simulink model "ALL_JP360_DBW_V6_5_1103"  (R2022a)
settings: Solver=FixedStepAuto  StartTime=0.0  StopTime=inf  FixedStep=0.01  RelTol=1e-3  EnableMultiTasking=on
model workspace (MAT data in the model file):
  g = 9.8
undefined symbols (not defined in the file or in its folder): canChannel, delta_v_p, IPM_Line_C0, IPM_Line_C1, IPM_Line_C2, IPM_Line_C3, M, M_p, MRR_ObjDistX, MRR_ObjDistY, MRR_ObjFusionCamID, MRR_ObjFusionSig, MRR_ObjID, MRR_ObjRelVelX, MRR_ObjRelVelY, MRR_ObjType, MRR_ObjUpdFlg, none, obj_vaild, untracktime, V, videoinput
libraries: canfdmsglib x230, canfdlib x76, slpidlib x24, simulink x18, dspstat3 x14, ctrlSharedLib x1, simulink_extras x1, imaqlib x1, realtime_pacer_lib x1, dspvision x1, visionsinks x1
(part 11 of 55)

== system ALL_JP360_DBW_V6_5_1103/MsgFromCAN/CCAN_ADCU_MsgFromCAN/CCAN_ADCU_GW_EMS_Tq_0x101 ==
  CCAN_ADCU_GW_EMS_Tq_0x101FromInData : Inport  OutDataTypeStr=Bus:CAN_FD_MESSAGE_BUS
  Bus Creator : BusCreator  Inputs=7  OutDataTypeStr=Bus:CCAN_ADCU_GW_EMS_Tq_0x101  NonVirtualBus=on
  CAN FD Unpack : canfdmsglib/CAN FD Unpack  CANdbFile=HiFire_JPT360_CCAN_Matrix_CAN_V1.72_VP_ADCU.dbc  MsgList=(none)  MsgName=GW_EMS_Tq_0x101  ProtocolMode=CAN FD  MsgIDType=Standard (11-bit identifier)  MsgIdentifier=257  MsgLength=8  SignalInfo={'Checksum_0x101','56','8','BE','unsigned','Standard','0','1','0','0','255';'EMS_EngSpeed','33','15','BE','unsigned','Standard','0','0.5','0','0','16383';'EMS_EngSpeedError','32','1','BE','unsigned','Standard','0','1','0','0','1';'EMS_IndicatedRealEngTorq','16','12','BE','unsigned','Standard','0','0.5','-1000','-1000','1000';'EMS_RngModTorqCrSLeadMax','12','12','BE','unsigned','Standard','0','0.5','-1000','-1000','1000';'EMS_RngModTorqCrSLeadMin','52','12','BE','unsigned','Standard','0','0.5','-1000','-1000','1000';'RollingCounter_0x101','48','4','BE','unsigned','Standard','0','1','0','0','15'}  IDPort=off  TimestampPort=off  ErrorPort=off  RemotePort=off  LengthPort=off  StatusPort=off  BRSPort=off  ESIPort=off  DLCPort=off  ApplyMinMax=off
      settings: SourceProductBaseCode=XP,ME,VN  DataFormat=CANdb specified signals
  Data Type Conversion1 : DataTypeConversion  OutDataTypeStr=uint8  SaturateOnIntegerOverflow=off  RndMeth=Floor
  Data Type Conversion{2,4..6} (4 alike) : DataTypeConversion  OutDataTypeStr=single  SaturateOnIntegerOverflow=off  RndMeth=Floor
  Data Type Conversion3 : DataTypeConversion  OutDataTypeStr=boolean  SaturateOnIntegerOverflow=off  RndMeth=Floor
  Data Type Conversion7 : DataTypeConversion  OutDataTypeStr=int8  SaturateOnIntegerOverflow=off  RndMeth=Floor
  CCAN_ADCU_GW_EMS_Tq_0x101FromOutData : Outport  OutDataTypeStr=Bus:CCAN_ADCU_GW_EMS_Tq_0x101
  wires:
  CAN FD Unpack/1 -> Data Type Conversion1/1
  CAN FD Unpack/2 -> Data Type Conversion2/1
  CAN FD Unpack/3 -> Data Type Conversion3/1
  CAN FD Unpack/4 -> Data Type Conversion4/1
  CAN FD Unpack/5 -> Data Type Conversion5/1
  CAN FD Unpack/6 -> Data Type Conversion6/1
  CAN FD Unpack/7 -> Data Type Conversion7/1
  Data Type Conversion1/1 -> Bus Creator/1  "Checksum_0x101"
  Data Type Conversion2/1 -> Bus Creator/2  "EMS_EngSpeed"
  Data Type Conversion3/1 -> Bus Creator/3  "EMS_EngSpeedError"
  Data Type Conversion4/1 -> Bus Creator/4  "EMS_IndicatedRealEngTorq"
  Data Type Conversion5/1 -> Bus Creator/5  "EMS_RngModTorqCrSLeadMax"
  Data Type Conversion6/1 -> Bus Creator/6  "EMS_RngModTorqCrSLeadMin"
  Data Type Conversion7/1 -> Bus Creator/7  "RollingCounter_0x101"
  Bus Creator/1 -> CCAN_ADCU_GW_EMS_Tq_0x101FromOutData/1  "CCAN_ADCU_GW_EMS_Tq_0x101FromOutData"
  CCAN_ADCU_GW_EMS_Tq_0x101FromInData/1 -> CAN FD Unpack/1  "CCAN_ADCU_GW_EMS_Tq_0x101FromInData"

== system ALL_JP360_DBW_V6_5_1103/MsgFromCAN/CCAN_ADCU_MsgFromCAN/CCAN_ADCU_GW_EMS_WhlTq_0x107 ==
  CCAN_ADCU_GW_EMS_WhlTq_0x107FromInData : Inport  OutDataTypeStr=Bus:CAN_FD_MESSAGE_BUS
  Bus Creator : BusCreator  Inputs=9  OutDataTypeStr=Bus:CCAN_ADCU_GW_EMS_WhlTq_0x107  NonVirtualBus=on
  CAN FD Unpack : canfdmsglib/CAN FD Unpack  CANdbFile=HiFire_JPT360_CCAN_Matrix_CAN_V1.72_VP_ADCU.dbc  MsgList=(none)  MsgName=GW_EMS_WhlTq_0x107  ProtocolMode=CAN FD  MsgIDType=Standard (11-bit identifier)  MsgIdentifier=263  MsgLength=8  SignalInfo={'Checksum_0x107','56','8','BE','unsigned','Standard','0','1','0','0','255';'EMS_ACCPedalRatioError','53','1','BE','unsigned','Standard','0','1','0','0','1';'EMS_AccPedalRatio','40','8','BE','unsigned','Standard','0','0.3937','0','0','99.9998';'EMS_AccRAWPedalRatio','32','8','BE','unsigned','Standard','0','0.3937','0','0','99.9998';'EMS_BrkPedalStasus','54','2','BE','unsigned','Standard','0','1','0','0','3';'EMS_KickDown','52','1','BE','unsigned','Standard','0','1','0','0','1';'MaxIndicatedTorqWhl','8','16','BE','unsigned','Standard','0','1','-30000','-30000','30000';'MinIndicatedTorqWhl','24','16','BE','unsigned','Standard','0','1','-30000','-30000','30000';'RollingCounter_0x107','48','4','BE','unsigned','Standard','0','1','0','0','15'}  IDPort=off  TimestampPort=off  ErrorPort=off  RemotePort=off  LengthPort=off  StatusPort=off  BRSPort=off  ESIPort=off  DLCPort=off  ApplyMinMax=off
      settings: SourceProductBaseCode=XP,ME,VN  DataFormat=CANdb specified signals
  Data Type Conversion1 : DataTypeConversion  OutDataTypeStr=uint8  SaturateOnIntegerOverflow=off  RndMeth=Floor
  Data Type Conversion2 : DataTypeConversion  OutDataTypeStr=boolean  SaturateOnIntegerOverflow=off  RndMeth=Floor
  Data Type Conversion3 : DataTypeConversion  OutDataTypeStr=single  SaturateOnIntegerOverflow=off  RndMeth=Floor
  Data Type Conversion4 : DataTypeConversion  OutDataTypeStr=single  SaturateOnIntegerOverflow=off  RndMeth=Floor
  Data Type Conversion5 : DataTypeConversion  OutDataTypeStr=int8  SaturateOnIntegerOverflow=off  RndMeth=Floor
  Data Type Conversion6 : DataTypeConversion  OutDataTypeStr=boolean  SaturateOnIntegerOverflow=off  RndMeth=Floor
  Data Type Conversion7 : DataTypeConversion  OutDataTypeStr=int16  SaturateOnIntegerOverflow=off  RndMeth=Floor
  Data Type Conversion8 : DataTypeConversion  OutDataTypeStr=int16  SaturateOnIntegerOverflow=off  RndMeth=Floor
  Data Type Conversion9 : DataTypeConversion  OutDataTypeStr=int8  SaturateOnIntegerOverflow=off  RndMeth=Floor
  CCAN_ADCU_GW_EMS_WhlTq_0x107FromOutData : Outport  OutDataTypeStr=Bus:CCAN_ADCU_GW_EMS_WhlTq_0x107
  wires:
  CAN FD Unpack/1 -> Data Type Conversion1/1
  CAN FD Unpack/2 -> Data Type Conversion2/1
  CAN FD Unpack/3 -> Data Type Conversion3/1
  CAN FD Unpack/4 -> Data Type Conversion4/1
  CAN FD Unpack/5 -> Data Type Conversion5/1
  CAN FD Unpack/6 -> Data Type Conversion6/1
  CAN FD Unpack/7 -> Data Type Conversion7/1
  CAN FD Unpack/8 -> Data Type Conversion8/1
  CAN FD Unpack/9 -> Data Type Conversion9/1
  Data Type Conversion1/1 -> Bus Creator/1  "Checksum_0x107"
  Data Type Conversion2/1 -> Bus Creator/2  "EMS_ACCPedalRatioError"
  Data Type Conversion3/1 -> Bus Creator/3  "EMS_AccPedalRatio"
  Data Type Conversion4/1 -> Bus Creator/4  "EMS_AccRAWPedalRatio"
  Data Type Conversion5/1 -> Bus Creator/5  "EMS_BrkPedalStasus"
  Data Type Conversion6/1 -> Bus Creator/6  "EMS_KickDown"
  Data Type Conversion7/1 -> Bus Creator/7  "MaxIndicatedTorqWhl"
  Data Type Conversion8/1 -> Bus Creator/8  "MinIndicatedTorqWhl"
  Data Type Conversion9/1 -> Bus Creator/9  "RollingCounter_0x107"
  Bus Creator/1 -> CCAN_ADCU_GW_EMS_WhlTq_0x107FromOutData/1  "CCAN_ADCU_GW_EMS_WhlTq_0x107FromOutData"
  CCAN_ADCU_GW_EMS_WhlTq_0x107FromInData/1 -> CAN FD Unpack/1  "CCAN_ADCU_GW_EMS_WhlTq_0x107FromInData"

== system ALL_JP360_DBW_V6_5_1103/MsgFromCAN/CCAN_ADCU_MsgFromCAN/CCAN_ADCU_GW_IC_0x510 ==
  CCAN_ADCU_GW_IC_0x510FromInData : Inport  OutDataTypeStr=Bus:CAN_FD_MESSAGE_BUS
  Bus Creator : BusCreator  Inputs=11  OutDataTypeStr=Bus:CCAN_ADCU_GW_IC_0x510  NonVirtualBus=on
  CAN FD Unpack : canfdmsglib/CAN FD Unpack  CANdbFile=HiFire_JPT360_CCAN_Matrix_CAN_V1.72_VP_ADCU.dbc  MsgList=(none)  MsgName=GW_IC_0x510  ProtocolMode=CAN FD  MsgIDType=Standard (11-bit identifier)  MsgIdentifier=1296  MsgLength=8  SignalInfo={'Checksum_0x510','56','8','BE','unsigned','Standard','0','1','0','0','255';'IC_AirbagTelltaleBehavior','38','3','BE','unsigned','Standard','0','1','0','0','7';'IC_BrakeAirPressure','53','8','BE','unsigned','Standard','0','30','0','0','1200';'IC_CabLockSts','52','1','BE','unsigned','Standard','0','1','0','0','1';'IC_DISFail','29','1','BE','unsigned','Standard','0','1','0','0','1';'IC_OdometerMasterValue','16','24','BE','unsigned','Standard','0','0.1','0','0','999999';'IC_QDashACCFail','30','2','BE','unsigned','Standard','0','1','0','0','3';'IC_VehBrkPump_ERR_IC','28','1','BE','unsigned','Standard','0','1','0','0','1';'IC_VehSpd_HMI','45','9','BE','unsigned','Standard','0','1','0','0','500';'IC_tirelearning','25','3','BE','unsigned','Standard','0','1','0','0','8';'RollingCounter_0x510','48','4','BE','unsigned','Standard','0','1','0','0','15'}  IDPort=off  TimestampPort=off  ErrorPort=off  RemotePort=off  LengthPort=off  StatusPort=off  BRSPort=off  ESIPort=off  DLCPort=off  ApplyMinMax=off
      settings: SourceProductBaseCode=XP,ME,VN  DataFormat=CANdb specified signals
  Data Type Conversion1 : DataTypeConversion  OutDataTypeStr=uint8  SaturateOnIntegerOverflow=off  RndMeth=Floor
  Data Type Conversion{2,7,10..11} (4 alike) : DataTypeConversion  OutDataTypeStr=int8  SaturateOnIntegerOverflow=off  RndMeth=Floor
  Data Type Conversion3 : DataTypeConversion  OutDataTypeStr=int16  SaturateOnIntegerOverflow=off  RndMeth=Floor
  Data Type Conversion4 : DataTypeConversion  OutDataTypeStr=boolean  SaturateOnIntegerOverflow=off  RndMeth=Floor
  Data Type Conversion5 : DataTypeConversion  OutDataTypeStr=boolean  SaturateOnIntegerOverflow=off  RndMeth=Floor
  Data Type Conversion6 : DataTypeConversion  OutDataTypeStr=single  SaturateOnIntegerOverflow=off  RndMeth=Floor
  Data Type Conversion8 : DataTypeConversion  OutDataTypeStr=boolean  SaturateOnIntegerOverflow=off  RndMeth=Floor
  Data Type Conversion9 : DataTypeConversion  OutDataTypeStr=int16  SaturateOnIntegerOverflow=off  RndMeth=Floor
  CCAN_ADCU_GW_IC_0x510FromOutData : Outport  OutDataTypeStr=Bus:CCAN_ADCU_GW_IC_0x510
  wires:
  CAN FD Unpack/1 -> Data Type Conversion1/1
  CAN FD Unpack/2 -> Data Type Conversion2/1
  CAN FD Unpack/3 -> Data Type Conversion3/1
  CAN FD Unpack/4 -> Data Type Conversion4/1
  CAN FD Unpack/5 -> Data Type Conversion5/1
  CAN FD Unpack/6 -> Data Type Conversion6/1
  CAN FD Unpack/7 -> Data Type Conversion7/1
  CAN FD Unpack/8 -> Data Type Conversion8/1
  CAN FD Unpack/9 -> Data Type Conversion9/1
  CAN FD Unpack/10 -> Data Type Conversion10/1
  CAN FD Unpack/11 -> Data Type Conversion11/1
  Data Type Conversion1/1 -> Bus Creator/1  "Checksum_0x510"
  Data Type Conversion2/1 -> Bus Creator/2  "IC_AirbagTelltaleBehavior"
  Data Type Conversion3/1 -> Bus Creator/3  "IC_BrakeAirPressure"
  Data Type Conversion4/1 -> Bus Creator/4  "IC_CabLockSts"
  Data Type Conversion5/1 -> Bus Creator/5  "IC_DISFail"
  Data Type Conversion6/1 -> Bus Creator/6  "IC_OdometerMasterValue"
  Data Type Conversion7/1 -> Bus Creator/7  "IC_QDashACCFail"
  Data Type Conversion8/1 -> Bus Creator/8  "IC_VehBrkPump_ERR_IC"
  Data Type Conversion9/1 -> Bus Creator/9  "IC_VehSpd_HMI"
  Data Type Conversion10/1 -> Bus Creator/10  "IC_tirelearning"
  Data Type Conversion11/1 -> Bus Creator/11  "RollingCounter_0x510"
  Bus Creator/1 -> CCAN_ADCU_GW_IC_0x510FromOutData/1  "CCAN_ADCU_GW_IC_0x510FromOutData"
  CCAN_ADCU_GW_IC_0x510FromInData/1 -> CAN FD Unpack/1  "CCAN_ADCU_GW_IC_0x510FromInData"

== system ALL_JP360_DBW_V6_5_1103/MsgFromCAN/CCAN_ADCU_MsgFromCAN/CCAN_ADCU_GW_IC_Time_0x581 ==
  CCAN_ADCU_GW_IC_Time_0x581FromInData : Inport  OutDataTypeStr=Bus:CAN_FD_MESSAGE_BUS
  Bus Creator : BusCreator  Inputs=6  OutDataTypeStr=Bus:CCAN_ADCU_GW_IC_Time_0x581  NonVirtualBus=on
  CAN FD Unpack : canfdmsglib/CAN FD Unpack  CANdbFile=HiFire_JPT360_CCAN_Matrix_CAN_V1.72_VP_ADCU.dbc  MsgList=(none)  MsgName=GW_IC_Time_0x581  ProtocolMode=CAN FD  MsgIDType=Standard (11-bit identifier)  MsgIdentifier=1409  MsgLength=8  SignalInfo={'IC_Date','16','8','BE','unsigned','Standard','0','1','1','1','31';'IC_Hour','24','8','BE','unsigned','Standard','0','1','0','0','23';'IC_Minute','32','8','BE','unsigned','Standard','0','1','0','0','59';'IC_Month','8','8','BE','unsigned','Standard','0','1','1','1','12';'IC_Second','40','8','BE','unsigned','Standard','0','1','0','0','59';'IC_Year','0','8','BE','unsigned','Standard','0','1','2017','2017','2272'}  IDPort=off  TimestampPort=off  ErrorPort=off  RemotePort=off  LengthPort=off  StatusPort=off  BRSPort=off  ESIPort=off  DLCPort=off  ApplyMinMax=off
      settings: SourceProductBaseCode=XP,ME,VN  DataFormat=CANdb specified signals
  Data Type Conversion{1..5} (5 alike) : DataTypeConversion  OutDataTypeStr=int8  SaturateOnIntegerOverflow=off  RndMeth=Floor
  Data Type Conversion6 : DataTypeConversion  OutDataTypeStr=int16  SaturateOnIntegerOverflow=off  RndMeth=Floor
  CCAN_ADCU_GW_IC_Time_0x581FromOutData : Outport  OutDataTypeStr=Bus:CCAN_ADCU_GW_IC_Time_0x581
  wires:
  CAN FD Unpack/1 -> Data Type Conversion1/1
  CAN FD Unpack/2 -> Data Type Conversion2/1
  CAN FD Unpack/3 -> Data Type Conversion3/1
  CAN FD Unpack/4 -> Data Type Conversion4/1
  CAN FD Unpack/5 -> Data Type Conversion5/1
  CAN FD Unpack/6 -> Data Type Conversion6/1
  Data Type Conversion1/1 -> Bus Creator/1  "IC_Date"
  Data Type Conversion2/1 -> Bus Creator/2  "IC_Hour"
  Data Type Conversion3/1 -> Bus Creator/3  "IC_Minute"
  Data Type Conversion4/1 -> Bus Creator/4  "IC_Month"
  Data Type Conversion5/1 -> Bus Creator/5  "IC_Second"
  Data Type Conversion6/1 -> Bus Creator/6  "IC_Year"
  Bus Creator/1 -> CCAN_ADCU_GW_IC_Time_0x581FromOutData/1  "CCAN_ADCU_GW_IC_Time_0x581FromOutData"
  CCAN_ADCU_GW_IC_Time_0x581FromInData/1 -> CAN FD Unpack/1  "CCAN_ADCU_GW_IC_Time_0x581FromInData"

== system ALL_JP360_DBW_V6_5_1103/MsgFromCAN/CCAN_ADCU_MsgFromCAN/CCAN_ADCU_GW_MP5_0x530 ==
  CCAN_ADCU_GW_MP5_0x530FromInData : Inport  OutDataTypeStr=Bus:CAN_FD_MESSAGE_BUS
  Bus Creator : BusCreator  Inputs=42  OutDataTypeStr=Bus:CCAN_ADCU_GW_MP5_0x530  NonVirtualBus=on
  CAN FD Unpack : canfdmsglib/CAN FD Unpack  CANdbFile=HiFire_JPT360_CCAN_Matrix_CAN_V1.72_VP_ADCU.dbc  MsgList=(none)  MsgName=GW_MP5_0x530  ProtocolMode=CAN FD  MsgIDType=Standard (11-bit identifier)  MsgIdentifier=1328  MsgLength=8  SignalInfo={'IVI_Driving_mode_req','36','4','BE','unsigned','Standard','0','1','0','0','15';'IVI_EcallRq','27','1','BE','unsigned','Standard','0','1','0','0','1';'IVI_FlashFlag','35','1','BE','unsigned','Standard','0','1','0','0','1';'IVI_HDCSwitchSetting','24','1','BE','unsigned','Standard','0','1','0','0','1';'MP5_AEB_ON_OFF','12','1','BE','unsigned','Standard','0','1','0','0','1';'MP5_AFS_SwtichSts','16','1','BE','unsigned','Standard','0','1','0','0','1';'MP5_APA_Available_Sts','56','2','BE','unsigned','Standard','0','1','0','0','1';'MP5_AVM_Angle','2','4','BE','unsigned','Standard','0','1','0','0','15';'MP5_AVM_Button','6','2','BE','unsigned','Standard','0','1','0','0','3';'MP5_AVM_RotationChange','63','6','BE','unsigned','Standard','0','1','0','0','63';'MP5_AVM_RotationDirection','61','2','BE','unsigned','Standard','0','1','0','0','3';'MP5_AlarmOrNot','23','1','BE','unsigned','Standard','0','1','0','0','1';'MP5_AlarmStatus','21','2','BE','unsigned','Standard','0','1','0','0','3';'MP5_BSDLCA_Active','41','1','BE','unsigned','Standard','0','1','0','0','1';'MP5_BSDSoundSwitchSts','32','1','BE','unsigned','Standard','0','1','0','0','1';'MP5_BSDSwitchSts','15','1','BE','unsigned','Standard','0','1','0','0','1';'MP5_CST_ON_OFF','33','1','BE','unsigned','Standard','0','1','0','0','1';'MP5_ConnectivityReset','34','1','BE','unsigned','Standard','0','1','0','0','1';'MP5_DCLC_switchSts','30','1','BE','unsigned','Standard','0','1','0','0','1';'MP5_DDDMenuReq','42','1','BE','unsigned','Standard','0','1','0','0','1';'MP5_DOA_Active','55','1','BE','unsigned','Standard','0','1','0','0','1';'MP5_ELK_switchSts','29','1','BE','unsigned','Standard','0','1','0','0','1';'MP5_ESP_ON_OFF','8','1','BE','unsigned','Standard','0','1','0','0','1';'MP5_EmergencyTowingSetting','25','1','BE','unsigned','Standard','0','1','0','0','1';'MP5_FCW_ON_OFF','13','1','BE','unsigned','Standard','0','1','0','0','1';'MP5_FCW_Sensitive','0','2','BE','unsigned','Standard','0','1','0','0','3';'MP5_ICMenuActive_Button','19','2','BE','unsigned','Standard','0','1','0','0','3';'MP5_ICMenuShift_Button','10','2','BE','unsigned','Standard','0','1','0','0','3';'MP5_IHCMenuReq','53','1','BE','unsigned','Standard','0','1','0','0','1';'MP5_LAEB_switchSts','28','1','BE','unsigned','Standard','0','1','0','0','1';'MP5_LDWSensitvity','46','2','BE','unsigned','Standard','0','1','0','0','3';'MP5_LDWWarning','44','2','BE','unsigned','Standard','0','1','0','0','3';'MP5_LaneAssitTypeReq','17','2','BE','unsigned','Standard','0','1','0','0','3';'MP5_PaakReset_Req','31','1','BE','unsigned','Standard','0','1','0','0','1';'MP5_PrdeProt_ON_OFF','54','1','BE','unsigned','Standard','0','1','0','0','1';'MP5_RCTA_Active','40','1','BE','unsigned','Standard','0','1','0','0','1';'MP5_RCW_Active','26','1','BE','unsigned','Standard','0','1','0','0','1';'MP5_SDGSwitchSts','14','1','BE','unsigned','Standard','0','1','0','0','1';'MP5_TPMSAutoLocationSetting','58','1','BE','unsigned','Standard','0','1','0','0','1';'MP5_TSRMenuReq','43','1','BE','unsigned','Standard','0','1','0','0','1';'MP5_View_Choice','9','1','BE','unsigned','Standard','0','1','0','0','1';'MP5_VspVoiceTypeSetting','59','2','BE','unsigned','Standard','0','1','0','0','3'}  IDPort=off  TimestampPort=off  ErrorPort=off  RemotePort=off  LengthPort=off  StatusPort=off  BRSPort=off  ESIPort=off  DLCPort=off  ApplyMinMax=off
      settings: SourceProductBaseCode=XP,ME,VN  DataFormat=CANdb specified signals
  Data Type Conversion{1,7..11,13,26..28,31..33,42} (14 alike) : DataTypeConversion  OutDataTypeStr=int8  SaturateOnIntegerOverflow=off  RndMeth=Floor
  Data Type Conversion{2..6,12,14..25,29..30,34..41} (28 alike) : DataTypeConversion  OutDataTypeStr=boolean  SaturateOnIntegerOverflow=off  RndMeth=Floor
  CCAN_ADCU_GW_MP5_0x530FromOutData : Outport  OutDataTypeStr=Bus:CCAN_ADCU_GW_MP5_0x530
  wires:
  CAN FD Unpack/1 -> Data Type Conversion1/1
  CAN FD Unpack/2 -> Data Type Conversion2/1
  CAN FD Unpack/3 -> Data Type Conversion3/1
  CAN FD Unpack/4 -> Data Type Conversion4/1
  CAN FD Unpack/5 -> Data Type Conversion5/1
  CAN FD Unpack/6 -> Data Type Conversion6/1
  CAN FD Unpack/7 -> Data Type Conversion7/1
  CAN FD Unpack/8 -> Data Type Conversion8/1
  CAN FD Unpack/9 -> Data Type Conversion9/1
  CAN FD Unpack/10 -> Data Type Conversion10/1
  CAN FD Unpack/11 -> Data Type Conversion11/1
  CAN FD Unpack/12 -> Data Type Conversion12/1
  CAN FD Unpack/13 -> Data Type Conversion13/1
  CAN FD Unpack/14 -> Data Type Conversion14/1
  CAN FD Unpack/15 -> Data Type Conversion15/1
  CAN FD Unpack/16 -> Data Type Conversion16/1
  CAN FD Unpack/17 -> Data Type Conversion17/1
  CAN FD Unpack/18 -> Data Type Conversion18/1
  CAN FD Unpack/19 -> Data Type Conversion19/1
  CAN FD Unpack/20 -> Data Type Conversion20/1
  CAN FD Unpack/21 -> Data Type Conversion21/1
  CAN FD Unpack/22 -> Data Type Conversion22/1
  CAN FD Unpack/23 -> Data Type Conversion23/1
  CAN FD Unpack/24 -> Data Type Conversion24/1
  CAN FD Unpack/25 -> Data Type Conversion25/1
  CAN FD Unpack/26 -> Data Type Conversion26/1
  CAN FD Unpack/27 -> Data Type Conversion27/1
  CAN FD Unpack/28 -> Data Type Conversion28/1
  CAN FD Unpack/29 -> Data Type Conversion29/1
  CAN FD Unpack/30 -> Data Type Conversion30/1
  CAN FD Unpack/31 -> Data Type Conversion31/1
  CAN FD Unpack/32 -> Data Type Conversion32/1
  CAN FD Unpack/33 -> Data Type Conversion33/1
  CAN FD Unpack/34 -> Data Type Conversion34/1
  CAN FD Unpack/35 -> Data Type Conversion35/1
  CAN FD Unpack/36 -> Data Type Conversion36/1
  CAN FD Unpack/37 -> Data Type Conversion37/1
  CAN FD Unpack/38 -> Data Type Conversion38/1
  CAN FD Unpack/39 -> Data Type Conversion39/1
  CAN FD Unpack/40 -> Data Type Conversion40/1
  CAN FD Unpack/41 -> Data Type Conversion41/1
  CAN FD Unpack/42 -> Data Type Conversion42/1
  Data Type Conversion1/1 -> Bus Creator/1  "IVI_Driving_mode_req"
  Data Type Conversion2/1 -> Bus Creator/2  "IVI_EcallRq"
  Data Type Conversion3/1 -> Bus Creator/3  "IVI_FlashFlag"
  Data Type Conversion4/1 -> Bus Creator/4  "IVI_HDCSwitchSetting"
  Data Type Conversion5/1 -> Bus Creator/5  "MP5_AEB_ON_OFF"
  Data Type Conversion6/1 -> Bus Creator/6  "MP5_AFS_SwtichSts"
  Data Type Conversion7/1 -> Bus Creator/7  "MP5_APA_Available_Sts"
  Data Type Conversion8/1 -> Bus Creator/8  "MP5_AVM_Angle"
  Data Type Conversion9/1 -> Bus Creator/9  "MP5_AVM_Button"
  Data Type Conversion10/1 -> Bus Creator/10  "MP5_AVM_RotationChange"
  Data Type Conversion11/1 -> Bus Creator/11  "MP5_AVM_RotationDirection"
  Data Type Conversion12/1 -> Bus Creator/12  "MP5_AlarmOrNot"
  Data Type Conversion13/1 -> Bus Creator/13  "MP5_AlarmStatus"
  Data Type Conversion14/1 -> Bus Creator/14  "MP5_BSDLCA_Active"
  Data Type Conversion15/1 -> Bus Creator/15  "MP5_BSDSoundSwitchSts"
  Data Type Conversion16/1 -> Bus Creator/16  "MP5_BSDSwitchSts"
  Data Type Conversion17/1 -> Bus Creator/17  "MP5_CST_ON_OFF"
  Data Type Conversion18/1 -> Bus Creator/18  "MP5_ConnectivityReset"
  Data Type Conversion19/1 -> Bus Creator/19  "MP5_DCLC_switchSts"
  Data Type Conversion20/1 -> Bus Creator/20  "MP5_DDDMenuReq"
  Data Type Conversion21/1 -> Bus Creator/21  "MP5_DOA_Active"
  Data Type Conversion22/1 -> Bus Creator/22  "MP5_ELK_switchSts"
  Data Type Conversion23/1 -> Bus Creator/23  "MP5_ESP_ON_OFF"
  Data Type Conversion24/1 -> Bus Creator/24  "MP5_EmergencyTowingSetting"
  Data Type Conversion25/1 -> Bus Creator/25  "MP5_FCW_ON_OFF"
  Data Type Conversion26/1 -> Bus Creator/26  "MP5_FCW_Sensitive"
  Data Type Conversion27/1 -> Bus Creator/27  "MP5_ICMenuActive_Button"
  Data Type Conversion28/1 -> Bus Creator/28  "MP5_ICMenuShift_Button"
  Data Type Conversion29/1 -> Bus Creator/29  "MP5_IHCMenuReq"
  Data Type Conversion30/1 -> Bus Creator/30  "MP5_LAEB_switchSts"
  Data Type Conversion31/1 -> Bus Creator/31  "MP5_LDWSensitvity"
  Data Type Conversion32/1 -> Bus Creator/32  "MP5_LDWWarning"
  Data Type Conversion33/1 -> Bus Creator/33  "MP5_LaneAssitTypeReq"
  Data Type Conversion34/1 -> Bus Creator/34  "MP5_PaakReset_Req"
  Data Type Conversion35/1 -> Bus Creator/35  "MP5_PrdeProt_ON_OFF"
  Data Type Conversion36/1 -> Bus Creator/36  "MP5_RCTA_Active"
  Data Type Conversion37/1 -> Bus Creator/37  "MP5_RCW_Active"
  Data Type Conversion38/1 -> Bus Creator/38  "MP5_SDGSwitchSts"
  Data Type Conversion39/1 -> Bus Creator/39  "MP5_TPMSAutoLocationSetting"
  Data Type Conversion40/1 -> Bus Creator/40  "MP5_TSRMenuReq"
  Data Type Conversion41/1 -> Bus Creator/41  "MP5_View_Choice"
  Data Type Conversion42/1 -> Bus Creator/42  "MP5_VspVoiceTypeSetting"
  Bus Creator/1 -> CCAN_ADCU_GW_MP5_0x530FromOutData/1  "CCAN_ADCU_GW_MP5_0x530FromOutData"
  CCAN_ADCU_GW_MP5_0x530FromInData/1 -> CAN FD Unpack/1  "CCAN_ADCU_GW_MP5_0x530FromInData"

== system ALL_JP360_DBW_V6_5_1103/MsgFromCAN/CCAN_ADCU_MsgFromCAN/CCAN_ADCU_GW_MP5_AVM_0x3A1 ==
  CCAN_ADCU_GW_MP5_AVM_0x3A1FromInData : Inport  OutDataTypeStr=Bus:CAN_FD_MESSAGE_BUS
  Bus Creator : BusCreator  Inputs=8  OutDataTypeStr=Bus:CCAN_ADCU_GW_MP5_AVM_0x3A1  NonVirtualBus=on
  CAN FD Unpack : canfdmsglib/CAN FD Unpack  CANdbFile=HiFire_JPT360_CCAN_Matrix_CAN_V1.72_VP_ADCU.dbc  MsgList=(none)  MsgName=GW_MP5_AVM_0x3A1  ProtocolMode=CAN FD  MsgIDType=Standard (11-bit identifier)  MsgIdentifier=929  MsgLength=8  SignalInfo={'MP5_AVMAuxLineCtrl','14','2','BE','unsigned','Standard','0','1','0','0','3';'MP5_AVMBodyColor','10','4','BE','unsigned','Standard','0','1','0','0','15';'MP5_AVMCarHyalineCtrl','0','8','BE','unsigned','Standard','0','1','0','0','100';'MP5_AVMRGearDlyDisplay','8','2','BE','unsigned','Standard','0','1','0','0','3';'MP5_InterfaceChangeSingnal','51','3','BE','unsigned','Standard','0','1','0','0','7';'MP5_TrnLfMode','54','2','BE','unsigned','Standard','0','1','0','0','3';'MP5_Xlevel','24','16','BE','unsigned','Standard','0','1','0','0','65534';'MP5_Ylevel','40','16','BE','unsigned','Standard','0','1','0','0','65534'}  IDPort=off  TimestampPort=off  ErrorPort=off  RemotePort=off  LengthPort=off  StatusPort=off  BRSPort=off  ESIPort=off  DLCPort=off  ApplyMinMax=off
      settings: SourceProductBaseCode=XP,ME,VN  DataFormat=CANdb specified signals
  Data Type Conversion{1..6} (6 alike) : DataTypeConversion  OutDataTypeStr=int8  SaturateOnIntegerOverflow=off  RndMeth=Floor
  Data Type Conversion7 : DataTypeConversion  OutDataTypeStr=uint16  SaturateOnIntegerOverflow=off  RndMeth=Floor
  Data Type Conversion8 : DataTypeConversion  OutDataTypeStr=uint16  SaturateOnIntegerOverflow=off  RndMeth=Floor
  CCAN_ADCU_GW_MP5_AVM_0x3A1FromOutData : Outport  OutDataTypeStr=Bus:CCAN_ADCU_GW_MP5_AVM_0x3A1
  wires:
  CAN FD Unpack/1 -> Data Type Conversion1/1
  CAN FD Unpack/2 -> Data Type Conversion2/1
  CAN FD Unpack/3 -> Data Type Conversion3/1
  CAN FD Unpack/4 -> Data Type Conversion4/1
  CAN FD Unpack/5 -> Data Type Conversion5/1
  CAN FD Unpack/6 -> Data Type Conversion6/1
  CAN FD Unpack/7 -> Data Type Conversion7/1
  CAN FD Unpack/8 -> Data Type Conversion8/1
  Data Type Conversion1/1 -> Bus Creator/1  "MP5_AVMAuxLineCtrl"
  Data Type Conversion2/1 -> Bus Creator/2  "MP5_AVMBodyColor"
  Data Type Conversion3/1 -> Bus Creator/3  "MP5_AVMCarHyalineCtrl"
  Data Type Conversion4/1 -> Bus Creator/4  "MP5_AVMRGearDlyDisplay"
  Data Type Conversion5/1 -> Bus Creator/5  "MP5_InterfaceChangeSingnal"
  Data Type Conversion6/1 -> Bus Creator/6  "MP5_TrnLfMode"
  Data Type Conversion7/1 -> Bus Creator/7  "MP5_Xlevel"
  Data Type Conversion8/1 -> Bus Creator/8  "MP5_Ylevel"
  Bus Creator/1 -> CCAN_ADCU_GW_MP5_AVM_0x3A1FromOutData/1  "CCAN_ADCU_GW_MP5_AVM_0x3A1FromOutData"
  CCAN_ADCU_GW_MP5_AVM_0x3A1FromInData/1 -> CAN FD Unpack/1  "CCAN_ADCU_GW_MP5_AVM_0x3A1FromInData"

== system ALL_JP360_DBW_V6_5_1103/MsgFromCAN/CCAN_ADCU_MsgFromCAN/CCAN_ADCU_GW_MP5_LicensePlateNum_0x375 ==
  CCAN_ADCU_GW_MP5_LicensePlateNum_0x375FromInData : Inport  OutDataTypeStr=Bus:CAN_FD_MESSAGE_BUS
  Bus Creator : BusCreator  Inputs=1  OutDataTypeStr=Bus:CCAN_ADCU_GW_MP5_LicensePlateNum_0x375  NonVirtualBus=on
  CAN FD Unpack : canfdmsglib/CAN FD Unpack  CANdbFile=HiFire_JPT360_CCAN_Matrix_CAN_V1.72_VP_ADCU.dbc  MsgList=(none)  MsgName=GW_MP5_LicensePlateNum_0x375  ProtocolMode=CAN FD  MsgIDType=Standard (11-bit identifier)  MsgIdentifier=885  MsgLength=8  SignalInfo={'MP5_LicenseInfo','56','64','BE','unsigned','Standard','0','1','0','0','1.84467440737095e+19'}  IDPort=off  TimestampPort=off  ErrorPort=off  RemotePort=off  LengthPort=off  StatusPort=off  BRSPort=off  ESIPort=off  DLCPort=off  ApplyMinMax=off
      settings: SourceProductBaseCode=XP,ME,VN  DataFormat=CANdb specified signals
  Data Type Conversion1 : DataTypeConversion  OutDataTypeStr=uint64  SaturateOnIntegerOverflow=off  RndMeth=Floor
  CCAN_ADCU_GW_MP5_LicensePlateNum_0x375FromOutData : Outport  OutDataTypeStr=Bus:CCAN_ADCU_GW_MP5_LicensePlateNum_0x375
  wires:
  Data Type Conversion1/1 -> Bus Creator/1  "MP5_LicenseInfo"
  Bus Creator/1 -> CCAN_ADCU_GW_MP5_LicensePlateNum_0x375FromOutData/1  "CCAN_ADCU_GW_MP5_LicensePlateNum_0x375FromOutData"
  CCAN_ADCU_GW_MP5_LicensePlateNum_0x375FromInData/1 -> CAN FD Unpack/1  "CCAN_ADCU_GW_MP5_LicensePlateNum_0x375FromInData"

== system ALL_JP360_DBW_V6_5_1103/MsgFromCAN/CCAN_ADCU_MsgFromCAN/CCAN_ADCU_GW_MP5_NAV_0x533 ==
  CCAN_ADCU_GW_MP5_NAV_0x533FromInData : Inport  OutDataTypeStr=Bus:CAN_FD_MESSAGE_BUS
  Bus Creator : BusCreator  Inputs=17  OutDataTypeStr=Bus:CCAN_ADCU_GW_MP5_NAV_0x533  NonVirtualBus=on
  CAN FD Unpack : canfdmsglib/CAN FD Unpack  CANdbFile=HiFire_JPT360_CCAN_Matrix_CAN_V1.72_VP_ADCU.dbc  MsgList=(none)  MsgName=GW_MP5_NAV_0x533  ProtocolMode=CAN FD  MsgIDType=Standard (11-bit identifier)  MsgIdentifier=1331  MsgLength=8  SignalInfo={'IVI_APA_SelPrkOutDirReq','34','3','BE','unsigned','Standard','0','1','0','0','7';'MP5_APAActive_Cmd','26','1','BE','unsigned','Standard','0','1','0','0','1';'MP5_APA_ConfirmButton','27','2','BE','unsigned','Standard','0','1','0','0','3';'MP5_APA_Function_Select','37','3','BE','unsigned','Standard','0','1','0','0','7';'MP5_ContnPrkgReq','24','2','BE','unsigned','Standard','0','1','0','0','3';'MP5_DSTSwReq','33','1','BE','unsigned','Standard','0','1','0','0','1';'MP5_FCTA_Active','44','1','BE','unsigned','Standard','0','1','0','0','1';'MP5_PwrSteeringModeReq','29','2','BE','unsigned','Standard','0','1','0','0','3';'MP5_RCTB_Active','45','1','BE','unsigned','Standard','0','1','0','0','1';'MP5_TrailerModeReq','46','2','BE','unsigned','Standard','0','1','0','0','3';'MP5_TrailerSMReq','32','1','BE','unsigned','Standard','0','1','0','0','1';'Nav_CountryCode','0','8','BE','unsigned','Standard','0','1','0','0','255';'Nav_CurrRoadType','12','4','BE','unsigned','Standard','0','1','0','0','15';'Nav_SpeedLimit','18','6','BE','unsigned','Standard','0','1','0','0','63';'Nav_SpeedLimitStatus','8','2','BE','unsigned','Standard','0','1','0','0','3';'Nav_SpeedLimitUnits','10','2','BE','unsigned','Standard','0','1','0','0','3';'Nav_Sts','31','1','BE','unsigned','Standard','0','1','0','0','1'}  IDPort=off  TimestampPort=off  ErrorPort=off  RemotePort=off  LengthPort=off  StatusPort=off  BRSPort=off  ESIPort=off  DLCPort=off  ApplyMinMax=off
      settings: SourceProductBaseCode=XP,ME,VN  DataFormat=CANdb specified signals
  Data Type Conversion{1,3..5,8,10,13..16} (10 alike) : DataTypeConversion  OutDataTypeStr=int8  SaturateOnIntegerOverflow=off  RndMeth=Floor
  Data Type Conversion{2,6..7,9,11,17} (6 alike) : DataTypeConversion  OutDataTypeStr=boolean  SaturateOnIntegerOverflow=off  RndMeth=Floor
  Data Type Conversion12 : DataTypeConversion  OutDataTypeStr=uint8  SaturateOnIntegerOverflow=off  RndMeth=Floor
  CCAN_ADCU_GW_MP5_NAV_0x533FromOutData : Outport  OutDataTypeStr=Bus:CCAN_ADCU_GW_MP5_NAV_0x533
  wires:
  CAN FD Unpack/1 -> Data Type Conversion1/1
  CAN FD Unpack/2 -> Data Type Conversion2/1
  CAN FD Unpack/3 -> Data Type Conversion3/1
  CAN FD Unpack/4 -> Data Type Conversion4/1
  CAN FD Unpack/5 -> Data Type Conversion5/1
  CAN FD Unpack/6 -> Data Type Conversion6/1
  CAN FD Unpack/7 -> Data Type Conversion7/1
  CAN FD Unpack/8 -> Data Type Conversion8/1
  CAN FD Unpack/9 -> Data Type Conversion9/1
  CAN FD Unpack/10 -> Data Type Conversion10/1
  CAN FD Unpack/11 -> Data Type Conversion11/1
  CAN FD Unpack/12 -> Data Type Conversion12/1
  CAN FD Unpack/13 -> Data Type Conversion13/1
  CAN FD Unpack/14 -> Data Type Conversion14/1
  CAN FD Unpack/15 -> Data Type Conversion15/1
  CAN FD Unpack/16 -> Data Type Conversion16/1
  CAN FD Unpack/17 -> Data Type Conversion17/1
  Data Type Conversion1/1 -> Bus Creator/1  "IVI_APA_SelPrkOutDirReq"
  Data Type Conversion2/1 -> Bus Creator/2  "MP5_APAActive_Cmd"
  Data Type Conversion3/1 -> Bus Creator/3  "MP5_APA_ConfirmButton"
  Data Type Conversion4/1 -> Bus Creator/4  "MP5_APA_Function_Select"
  Data Type Conversion5/1 -> Bus Creator/5  "MP5_ContnPrkgReq"
  Data Type Conversion6/1 -> Bus Creator/6  "MP5_DSTSwReq"
  Data Type Conversion7/1 -> Bus Creator/7  "MP5_FCTA_Active"
  Data Type Conversion8/1 -> Bus Creator/8  "MP5_PwrSteeringModeReq"
  Data Type Conversion9/1 -> Bus Creator/9  "MP5_RCTB_Active"
  Data Type Conversion10/1 -> Bus Creator/10  "MP5_TrailerModeReq"
  Data Type Conversion11/1 -> Bus Creator/11  "MP5_TrailerSMReq"
  Data Type Conversion12/1 -> Bus Creator/12  "Nav_CountryCode"
  Data Type Conversion13/1 -> Bus Creator/13  "Nav_CurrRoadType"
  Data Type Conversion14/1 -> Bus Creator/14  "Nav_SpeedLimit"
  Data Type Conversion15/1 -> Bus Creator/15  "Nav_SpeedLimitStatus"
  Data Type Conversion16/1 -> Bus Creator/16  "Nav_SpeedLimitUnits"
  Data Type Conversion17/1 -> Bus Creator/17  "Nav_Sts"
  Bus Creator/1 -> CCAN_ADCU_GW_MP5_NAV_0x533FromOutData/1  "CCAN_ADCU_GW_MP5_NAV_0x533FromOutData"
  CCAN_ADCU_GW_MP5_NAV_0x533FromInData/1 -> CAN FD Unpack/1  "CCAN_ADCU_GW_MP5_NAV_0x533FromInData"

== system ALL_JP360_DBW_V6_5_1103/MsgFromCAN/CCAN_ADCU_MsgFromCAN/CCAN_ADCU_GW_SRS_0x350 ==
  CCAN_ADCU_GW_SRS_0x350FromInData : Inport  OutDataTypeStr=Bus:CAN_FD_MESSAGE_BUS
  Bus Creator : BusCreator  Inputs=9  OutDataTypeStr=Bus:CCAN_ADCU_GW_SRS_0x350  NonVirtualBus=on
  CAN FD Unpack : canfdmsglib/CAN FD Unpack  CANdbFile=HiFire_JPT360_CCAN_Matrix_CAN_V1.72_VP_ADCU.dbc  MsgList=(none)  MsgName=GW_SRS_0x350  ProtocolMode=CAN FD  MsgIDType=Standard (11-bit identifier)  MsgIdentifier=848  MsgLength=8  SignalInfo={'Checksum_0x350','56','8','BE','unsigned','Standard','0','1','0','0','255';'RollingCounter_0x350','48','4','BE','unsigned','Standard','0','1','0','0','15';'SRS_AirBagFailSts','23','2','BE','unsigned','Standard','0','1','0','0','3';'SRS_CrashOutputSts','7','1','BE','unsigned','Standard','0','1','0','0','1';'SRS_SBR_Driver','5','2','BE','unsigned','Standard','0','1','0','0','3';'SRS_SBR_Passenger','3','2','BE','unsigned','Standard','0','1','0','0','3';'SRS_SBR_SecondRowLeft','14','2','BE','unsigned','Standard','0','1','0','0','3';'SRS_SBR_SecondRowMid','12','2','BE','unsigned','Standard','0','1','0','0','3';'SRS_SBR_SecondRowRight','10','2','BE','unsigned','Standard','0','1','0','0','3'}  IDPort=off  TimestampPort=off  ErrorPort=off  RemotePort=off  LengthPort=off  StatusPort=off  BRSPort=off  ESIPort=off  DLCPort=off  ApplyMinMax=off
      settings: SourceProductBaseCode=XP,ME,VN  DataFormat=CANdb specified signals
  Data Type Conversion1 : DataTypeConversion  OutDataTypeStr=uint8  SaturateOnIntegerOverflow=off  RndMeth=Floor
  Data Type Conversion{2..3,5..9} (7 alike) : DataTypeConversion  OutDataTypeStr=int8  SaturateOnIntegerOverflow=off  RndMeth=Floor
  Data Type Conversion4 : DataTypeConversion  OutDataTypeStr=boolean  SaturateOnIntegerOverflow=off  RndMeth=Floor
  CCAN_ADCU_GW_SRS_0x350FromOutData : Outport  OutDataTypeStr=Bus:CCAN_ADCU_GW_SRS_0x350
  wires:
  CAN FD Unpack/1 -> Data Type Conversion1/1
  CAN FD Unpack/2 -> Data Type Conversion2/1
  CAN FD Unpack/3 -> Data Type Conversion3/1
  CAN FD Unpack/4 -> Data Type Conversion4/1
  CAN FD Unpack/5 -> Data Type Conversion5/1
  CAN FD Unpack/6 -> Data Type Conversion6/1
  CAN FD Unpack/7 -> Data Type Conversion7/1
  CAN FD Unpack/8 -> Data Type Conversion8/1
  CAN FD Unpack/9 -> Data Type Conversion9/1
  Data Type Conversion1/1 -> Bus Creator/1  "Checksum_0x350"
  Data Type Conversion2/1 -> Bus Creator/2  "RollingCounter_0x350"
  Data Type Conversion3/1 -> Bus Creator/3  "SRS_AirBagFailSts"
  Data Type Conversion4/1 -> Bus Creator/4  "SRS_CrashOutputSts"
  Data Type Conversion5/1 -> Bus Creator/5  "SRS_SBR_Driver"
  Data Type Conversion6/1 -> Bus Creator/6  "SRS_SBR_Passenger"
  Data Type Conversion7/1 -> Bus Creator/7  "SRS_SBR_SecondRowLeft"
  Data Type Conversion8/1 -> Bus Creator/8  "SRS_SBR_SecondRowMid"
  Data Type Conversion9/1 -> Bus Creator/9  "SRS_SBR_SecondRowRight"
  Bus Creator/1 -> CCAN_ADCU_GW_SRS_0x350FromOutData/1  "CCAN_ADCU_GW_SRS_0x350FromOutData"
  CCAN_ADCU_GW_SRS_0x350FromInData/1 -> CAN FD Unpack/1  "CCAN_ADCU_GW_SRS_0x350FromInData"

== system ALL_JP360_DBW_V6_5_1103/MsgFromCAN/CCAN_ADCU_MsgFromCAN/CCAN_ADCU_GW_TCU_GearInfo_0x123 ==
  CCAN_ADCU_GW_TCU_GearInfo_0x123FromInData : Inport  OutDataTypeStr=Bus:CAN_FD_MESSAGE_BUS
  Bus Creator : BusCreator  Inputs=20  OutDataTypeStr=Bus:CCAN_ADCU_GW_TCU_GearInfo_0x123  NonVirtualBus=on
  CAN FD Unpack : canfdmsglib/CAN FD Unpack  CANdbFile=HiFire_JPT360_CCAN_Matrix_CAN_V1.72_VP_ADCU.dbc  MsgList=(none)  MsgName=GW_TCU_GearInfo_0x123  ProtocolMode=CAN FD  MsgIDType=Standard (11-bit identifier)  MsgIdentifier=291  MsgLength=8  SignalInfo={'Checksum_0x123','56','8','BE','unsigned','Standard','0','1','0','0','255';'RollingCounter_0x123','48','4','BE','unsigned','Standard','0','1','0','0','15';'ShiftLeverPos_SBWM','21','3','BE','unsigned','Standard','0','1','0','0','7';'TCU_CurrentGearPosition','4','4','BE','unsigned','Standard','0','1','0','0','15';'TCU_DisplayGear','8','4','BE','unsigned','Standard','0','1','0','0','15';'TCU_DriverIntervention','33','1','BE','unsigned','Standard','0','1','0','0','1';'TCU_DrivingModeChange_Fault_flag','46','1','BE','unsigned','Standard','0','1','0','0','1';'TCU_Driving_mode_req','40','4','BE','unsigned','Standard','0','1','0','0','15';'TCU_EPBLockReq','44','1','BE','unsigned','Standard','0','1','0','0','1';'TCU_GearSelectorReq','12','4','BE','unsigned','Standard','0','1','0','0','15';'TCU_GearShiftInProgress','20','1','BE','unsigned','Standard','0','1','0','0','1';'TCU_OverallRatio','24','11','BE','unsigned','Standard','0','0.01','0','0','20';'TCU_ShiftLevertoPReq','54','2','BE','unsigned','Standard','0','1','0','0','3';'TCU_ShiftLevertoPReqInvalid','47','1','BE','unsigned','Standard','0','1','0','0','1';'TCU_StGearMode','36','4','BE','unsigned','Standard','0','1','0','0','15';'TCU_TargetGearReq','0','4','BE','unsigned','Standard','0','1','0','0','15';'TCU_TrsmFaultFlag','34','2','BE','unsigned','Standard','0','1','0','0','3';'TCU_available','32','1','BE','unsigned','Standard','0','1','0','0','1';'TCU_highresistance','45','1','BE','unsigned','Standard','0','1','0','0','1';'TCU_transPmotorparkReq','52','2','BE','unsigned','Standard','0','1','0','0','3'}  IDPort=off  TimestampPort=off  ErrorPort=off  RemotePort=off  LengthPort=off  StatusPort=off  BRSPort=off  ESIPort=off  DLCPort=off  ApplyMinMax=off
      settings: SourceProductBaseCode=XP,ME,VN  DataFormat=CANdb specified signals
  Data Type Conversion1 : DataTypeConversion  OutDataTypeStr=uint8  SaturateOnIntegerOverflow=off  RndMeth=Floor
  Data Type Conversion{2..5,8,10,13,15..17,20} (11 alike) : DataTypeConversion  OutDataTypeStr=int8  SaturateOnIntegerOverflow=off  RndMeth=Floor
  Data Type Conversion{6..7,9,11,14,18..19} (7 alike) : DataTypeConversion  OutDataTypeStr=boolean  SaturateOnIntegerOverflow=off  RndMeth=Floor
  Data Type Conversion12 : DataTypeConversion  OutDataTypeStr=single  SaturateOnIntegerOverflow=off  RndMeth=Floor
  CCAN_ADCU_GW_TCU_GearInfo_0x123FromOutData : Outport  OutDataTypeStr=Bus:CCAN_ADCU_GW_TCU_GearInfo_0x123
  wires:
  CAN FD Unpack/1 -> Data Type Conversion1/1
  CAN FD Unpack/2 -> Data Type Conversion2/1
  CAN FD Unpack/3 -> Data Type Conversion3/1
  CAN FD Unpack/4 -> Data Type Conversion4/1
  CAN FD Unpack/5 -> Data Type Conversion5/1
  CAN FD Unpack/6 -> Data Type Conversion6/1
  CAN FD Unpack/7 -> Data Type Conversion7/1
  CAN FD Unpack/8 -> Data Type Conversion8/1
  CAN FD Unpack/9 -> Data Type Conversion9/1
  CAN FD Unpack/10 -> Data Type Conversion10/1
  CAN FD Unpack/11 -> Data Type Conversion11/1
  CAN FD Unpack/12 -> Data Type Conversion12/1
  CAN FD Unpack/13 -> Data Type Conversion13/1
  CAN FD Unpack/14 -> Data Type Conversion14/1
  CAN FD Unpack/15 -> Data Type Conversion15/1
  CAN FD Unpack/16 -> Data Type Conversion16/1
  CAN FD Unpack/17 -> Data Type Conversion17/1
  CAN FD Unpack/18 -> Data Type Conversion18/1
  CAN FD Unpack/19 -> Data Type Conversion19/1
  CAN FD Unpack/20 -> Data Type Conversion20/1
  Data Type Conversion1/1 -> Bus Creator/1  "Checksum_0x123"
  Data Type Conversion2/1 -> Bus Creator/2  "RollingCounter_0x123"
  Data Type Conversion3/1 -> Bus Creator/3  "ShiftLeverPos_SBWM"
  Data Type Conversion4/1 -> Bus Creator/4  "TCU_CurrentGearPosition"
  Data Type Conversion5/1 -> Bus Creator/5  "TCU_DisplayGear"
  Data Type Conversion6/1 -> Bus Creator/6  "TCU_DriverIntervention"
  Data Type Conversion7/1 -> Bus Creator/7  "TCU_DrivingModeChange_Fault_flag"
  Data Type Conversion8/1 -> Bus Creator/8  "TCU_Driving_mode_req"
  Data Type Conversion9/1 -> Bus Creator/9  "TCU_EPBLockReq"
  Data Type Conversion10/1 -> Bus Creator/10  "TCU_GearSelectorReq"
  Data Type Conversion11/1 -> Bus Creator/11  "TCU_GearShiftInProgress"
  Data Type Conversion12/1 -> Bus Creator/12  "TCU_OverallRatio"
  Data Type Conversion13/1 -> Bus Creator/13  "TCU_ShiftLevertoPReq"
  Data Type Conversion14/1 -> Bus Creator/14  "TCU_ShiftLevertoPReqInvalid"
  Data Type Conversion15/1 -> Bus Creator/15  "TCU_StGearMode"
  Data Type Conversion16/1 -> Bus Creator/16  "TCU_TargetGearReq"
  Data Type Conversion17/1 -> Bus Creator/17  "TCU_TrsmFaultFlag"
  Data Type Conversion18/1 -> Bus Creator/18  "TCU_available"
  Data Type Conversion19/1 -> Bus Creator/19  "TCU_highresistance"
  Data Type Conversion20/1 -> Bus Creator/20  "TCU_transPmotorparkReq"
  Bus Creator/1 -> CCAN_ADCU_GW_TCU_GearInfo_0x123FromOutData/1  "CCAN_ADCU_GW_TCU_GearInfo_0x123FromOutData"
  CCAN_ADCU_GW_TCU_GearInfo_0x123FromInData/1 -> CAN FD Unpack/1  "CCAN_ADCU_GW_TCU_GearInfo_0x123FromInData"

== system ALL_JP360_DBW_V6_5_1103/MsgFromCAN/CCAN_ADCU_MsgFromCAN/CCAN_ADCU_SAS_Sensor_0x175 ==
  CCAN_ADCU_SAS_Sensor_0x175FromInData : Inport  OutDataTypeStr=Bus:CAN_FD_MESSAGE_BUS
  Bus Creator : BusCreator  Inputs=10  OutDataTypeStr=Bus:CCAN_ADCU_SAS_Sensor_0x175  NonVirtualBus=on
  CAN FD Unpack : canfdmsglib/CAN FD Unpack  CANdbFile=HiFire_JPT360_CCAN_Matrix_CAN_V1.72_VP_ADCU.dbc  MsgList=(none)  MsgName=SAS_Sensor_0x175  ProtocolMode=CAN FD  MsgIDType=Standard (11-bit identifier)  MsgIdentifier=373  MsgLength=8  SignalInfo={'Checksum_0x175','56','8','BE','unsigned','Standard','0','1','0','0','255';'RollingCounter_0x175','48','4','BE','unsigned','Standard','0','1','0','0','15';'SAS_Raw_SASStsSnsr','54','1','BE','unsigned','Standard','0','1','0','0','1';'SAS_Raw_SteerWheelAngle','24','16','BE','unsigned','Standard','0','0.0238','-780','-780','779.7';'SAS_SASStsCal','53','1','BE','unsigned','Standard','0','1','0','0','1';'SAS_SASStsSnsr','55','1','BE','unsigned','Standard','0','1','0','0','1';'SAS_SteerWheelAngle','8','16','BE','unsigned','Standard','0','0.0238','-780','-780','779.7';'SAS_SteerWheelRotSpd','42','14','BE','unsigned','Standard','0','0.125','-1024','-1024','1023.75';'SAS_SteerWheelRotSpdStatus','41','1','BE','unsigned','Standard','0','1','0','0','1';'SAS_TrimmingSts','40','1','BE','unsigned','Standard','0','1','0','0','1'}  IDPort=off  TimestampPort=off  ErrorPort=off  RemotePort=off  LengthPort=off  StatusPort=off  BRSPort=off  ESIPort=off  DLCPort=off  ApplyMinMax=off
      settings: SourceProductBaseCode=XP,ME,VN  DataFormat=CANdb specified signals
  Data Type Conversion1 : DataTypeConversion  OutDataTypeStr=uint8  SaturateOnIntegerOverflow=off  RndMeth=Floor
  Data Type Conversion{3,5..6,9..10} (5 alike) : DataTypeConversion  OutDataTypeStr=boolean  SaturateOnIntegerOverflow=off  RndMeth=Floor
  Data Type Conversion2 : DataTypeConversion  OutDataTypeStr=int8  SaturateOnIntegerOverflow=off  RndMeth=Floor
  Data Type Conversion4 : DataTypeConversion  OutDataTypeStr=single  SaturateOnIntegerOverflow=off  RndMeth=Floor
  Data Type Conversion7 : DataTypeConversion  OutDataTypeStr=single  SaturateOnIntegerOverflow=off  RndMeth=Floor
  Data Type Conversion8 : DataTypeConversion  OutDataTypeStr=single  SaturateOnIntegerOverflow=off  RndMeth=Floor
  CCAN_ADCU_SAS_Sensor_0x175FromOutData : Outport  OutDataTypeStr=Bus:CCAN_ADCU_SAS_Sensor_0x175
  wires:
  CAN FD Unpack/1 -> Data Type Conversion1/1
  CAN FD Unpack/2 -> Data Type Conversion2/1
  CAN FD Unpack/3 -> Data Type Conversion3/1
  CAN FD Unpack/4 -> Data Type Conversion4/1
  CAN FD Unpack/5 -> Data Type Conversion5/1
  CAN FD Unpack/6 -> Data Type Conversion6/1
  CAN FD Unpack/7 -> Data Type Conversion7/1
  CAN FD Unpack/8 -> Data Type Conversion8/1
  CAN FD Unpack/9 -> Data Type Conversion9/1
  CAN FD Unpack/10 -> Data Type Conversion10/1
  Data Type Conversion1/1 -> Bus Creator/1  "Checksum_0x175"
  Data Type Conversion2/1 -> Bus Creator/2  "RollingCounter_0x175"
  Data Type Conversion3/1 -> Bus Creator/3  "SAS_Raw_SASStsSnsr"
  Data Type Conversion4/1 -> Bus Creator/4  "SAS_Raw_SteerWheelAngle"
  Data Type Conversion5/1 -> Bus Creator/5  "SAS_SASStsCal"
  Data Type Conversion6/1 -> Bus Creator/6  "SAS_SASStsSnsr"
  Data Type Conversion7/1 -> Bus Creator/7  "SAS_SteerWheelAngle"
  Data Type Conversion8/1 -> Bus Creator/8  "SAS_SteerWheelRotSpd"
  Data Type Conversion9/1 -> Bus Creator/9  "SAS_SteerWheelRotSpdStatus"
  Data Type Conversion10/1 -> Bus Creator/10  "SAS_TrimmingSts"
  Bus Creator/1 -> CCAN_ADCU_SAS_Sensor_0x175FromOutData/1  "CCAN_ADCU_SAS_Sensor_0x175FromOutData"
  CCAN_ADCU_SAS_Sensor_0x175FromInData/1 -> CAN FD Unpack/1  "CCAN_ADCU_SAS_Sensor_0x175FromInData"

== system ALL_JP360_DBW_V6_5_1103/MsgFromCAN/CCAN_ADCU_MsgFromCAN/CCAN_ADCU_SRR_FL_0x27B ==
  CCAN_ADCU_SRR_FL_0x27BFromInData : Inport  OutDataTypeStr=Bus:CAN_FD_MESSAGE_BUS
  Bus Creator : BusCreator  Inputs=8  OutDataTypeStr=Bus:CCAN_ADCU_SRR_FL_0x27B  NonVirtualBus=on
  CAN FD Unpack : canfdmsglib/CAN FD Unpack  CANdbFile=HiFire_JPT360_CCAN_Matrix_CAN_V1.72_VP_ADCU.dbc  MsgList=(none)  MsgName=SRR_FL_0x27B  ProtocolMode=CAN FD  MsgIDType=Standard (11-bit identifier)  MsgIdentifier=635  MsgLength=8  SignalInfo={'BSD_FCTA_Active','0','2','BE','unsigned','Standard','0','1','0','0','3';'BSD_FCTA_State','7','1','BE','unsigned','Standard','0','1','0','0','1';'BSD_FCTA_display','12','4','BE','unsigned','Standard','0','1','0','0','15';'Checksum_0x27B','56','8','BE','unsigned','Standard','0','1','0','0','255';'FCTA_OFFTelltale','6','1','BE','unsigned','Standard','0','1','0','0','1';'FCTA_warningReqLeft','4','2','BE','unsigned','Standard','0','1','0','0','3';'FCTA_warningReqRight','2','2','BE','unsigned','Standard','0','1','0','0','3';'RollingCounter_0x27B','48','4','BE','unsigned','Standard','0','1','0','0','15'}  IDPort=off  TimestampPort=off  ErrorPort=off  RemotePort=off  LengthPort=off  StatusPort=off  BRSPort=off  ESIPort=off  DLCPort=off  ApplyMinMax=off
      settings: SourceProductBaseCode=XP,ME,VN  DataFormat=CANdb specified signals
  Data Type Conversion{1,3,6..8} (5 alike) : DataTypeConversion  OutDataTypeStr=int8  SaturateOnIntegerOverflow=off  RndMeth=Floor
  Data Type Conversion2 : DataTypeConversion  OutDataTypeStr=boolean  SaturateOnIntegerOverflow=off  RndMeth=Floor
  Data Type Conversion4 : DataTypeConversion  OutDataTypeStr=uint8  SaturateOnIntegerOverflow=off  RndMeth=Floor
  Data Type Conversion5 : DataTypeConversion  OutDataTypeStr=boolean  SaturateOnIntegerOverflow=off  RndMeth=Floor
  CCAN_ADCU_SRR_FL_0x27BFromOutData : Outport  OutDataTypeStr=Bus:CCAN_ADCU_SRR_FL_0x27B
  wires:
  CAN FD Unpack/1 -> Data Type Conversion1/1
  CAN FD Unpack/2 -> Data Type Conversion2/1
  CAN FD Unpack/3 -> Data Type Conversion3/1
  CAN FD Unpack/4 -> Data Type Conversion4/1
  CAN FD Unpack/5 -> Data Type Conversion5/1
  CAN FD Unpack/6 -> Data Type Conversion6/1
  CAN FD Unpack/7 -> Data Type Conversion7/1
  CAN FD Unpack/8 -> Data Type Conversion8/1
  Data Type Conversion1/1 -> Bus Creator/1  "BSD_FCTA_Active"
  Data Type Conversion2/1 -> Bus Creator/2  "BSD_FCTA_State"
  Data Type Conversion3/1 -> Bus Creator/3  "BSD_FCTA_display"
  Data Type Conversion4/1 -> Bus Creator/4  "Checksum_0x27B"
  Data Type Conversion5/1 -> Bus Creator/5  "FCTA_OFFTelltale"
  Data Type Conversion6/1 -> Bus Creator/6  "FCTA_warningReqLeft"
  Data Type Conversion7/1 -> Bus Creator/7  "FCTA_warningReqRight"
  Data Type Conversion8/1 -> Bus Creator/8  "RollingCounter_0x27B"
  Bus Creator/1 -> CCAN_ADCU_SRR_FL_0x27BFromOutData/1  "CCAN_ADCU_SRR_FL_0x27BFromOutData"
  CCAN_ADCU_SRR_FL_0x27BFromInData/1 -> CAN FD Unpack/1  "CCAN_ADCU_SRR_FL_0x27BFromInData"
